simulink model "lookupTableDynamic_TestGen31"  (R2017b)
settings: Solver=FixedStepDiscrete  StartTime=0.0  StopTime=10.0  RelTol=1e-3
libraries: simulink x1
settings Model: Creator=ktrinh  LastModifiedBy=ktrinh
settings DebuggingCC: ParameterOverflowMsg=none

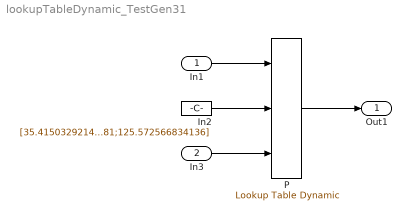
== system lookupTableDynamic_TestGen31 ==
  In1 : Inport  OutMin=33.415  OutMax=128  OutDataTypeStr=int32  PortDimensions=[2,3]
  In3 : Inport  Port=2  PortDimensions=5
  In2 : Constant  Value=[35.4150329214313;38.0933456216653;51.5084750834238;55.1015161619581;125.572566834136]  OutDataTypeStr=int32
  P : simulink/Lookup Tables/Lookup Table Dynamic  LookUpMeth=Use Input Below  OutDataType=fixdt('uint8')  OutScaling=[]  OutputDataTypeScalingMode=Specify via dialog  OutDataTypeStr=uint8  RndMeth=Nearest  DoSatur=on
      settings: SourceProductName=Simulink
  Out1 : Outport
  wires:
  In1/1 -> P/1
  In2/1 -> P/2
  In3/1 -> P/3
  P/1 -> Out1/1
